simulink model "sampleModel307"  (R2021b)
settings: Solver=VariableStepAuto  StartTime=0.0  StopTime=10.0  RelTol=1e-3
libraries: simulink x3
settings Model: Creator=user  LastModifiedBy=user

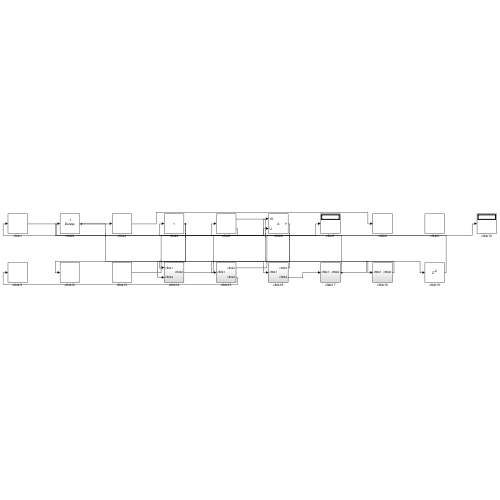
[thumbnail: Simulink's stored preview of the top-level diagram]
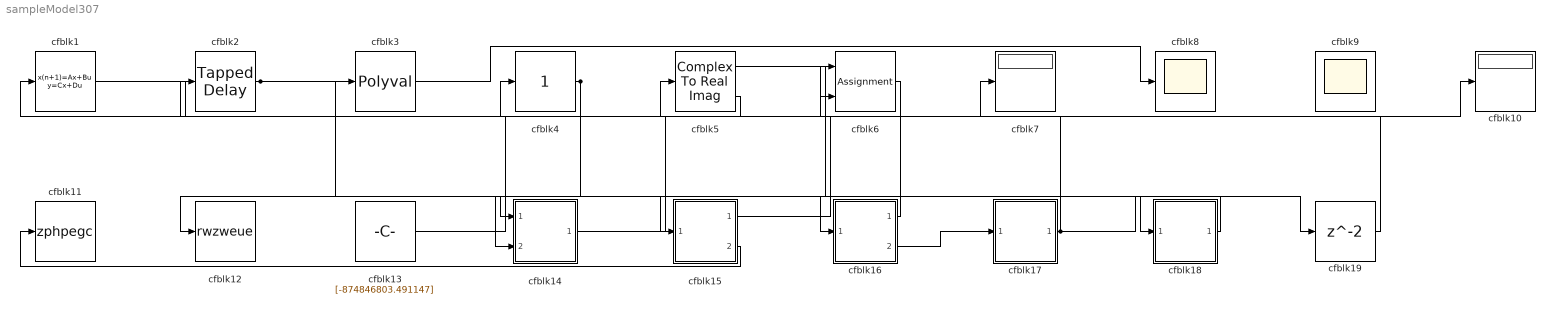
== system sampleModel307 ==
  cfblk1 : DiscreteStateSpace
  cfblk10 : Display
  cfblk11 : ToWorkspace  VariableName=zphpegc  SaveFormat=Timeseries  SampleTime=-1
  cfblk12 : ToWorkspace  VariableName=rwzweue  SaveFormat=Timeseries  SampleTime=-1
  cfblk13 : Constant  Value=[-874846803.491147]  SampleTime=1
  cfblk14 : Subsystem
  cfblk15 : Subsystem
  cfblk16 : Subsystem
  cfblk17 : Subsystem
  cfblk18 : Subsystem
  cfblk19 : Delay  SampleTime=1
  cfblk2 : simulink/Discrete/Tapped Delay  vinit=0.0  samptime=-1  NumDelays=1  DelayOrder=Oldest  includeCurrent=off
  cfblk3 : Polyval  Coefs=[ +2.081618890e-019, -1.441693666e-014, +4.719686976e-010, -8.536869453e-006, +1.621573104e-001, -8.087801117e+001 ]
  cfblk4 : simulink/Math Operations/Slider Gain  gain=1  low=0  high=2
  cfblk5 : ComplexToRealImag
  cfblk6 : Assignment  DiagnosticForDimensions=Warning  IndexOptions=Index vector (dialog)  Indices=1  OutputSizes=1
  cfblk7 : Display
  cfblk8 : Scope
  cfblk9 : Scope
      settings: Floating=on
  wires:
  cfblk4/1 -> cfblk12/1, cfblk14/2(cfblk4)
  cfblk14/1(cfblk2) -> cfblk10/1
  cfblk17/1(cfblk2) -> cfblk4/1, cfblk19/1
  cfblk5/1 -> cfblk18/1(cfblk1)
  cfblk16/1(cfblk2) -> cfblk5/1
  cfblk15/1(cfblk2) -> cfblk7/1
  cfblk5/2 -> cfblk1/1
  cfblk3/1 -> cfblk8/1
  cfblk15/2(cfblk4) -> cfblk11/1
  cfblk13/1 -> cfblk6/1
  cfblk2/1 -> cfblk3/1, cfblk16/1(cfblk1)
  cfblk1/1 -> cfblk6/2
  cfblk6/1 -> cfblk15/1(cfblk1)
  cfblk18/1(cfblk2) -> cfblk14/1(cfblk1)
  cfblk16/2(cfblk4) -> cfblk17/1(cfblk1)
  cfblk19/1 -> cfblk2/1

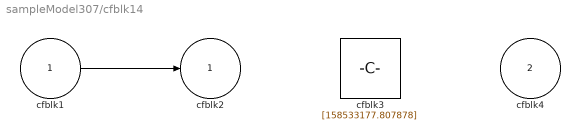
== system sampleModel307/cfblk14 ==
  cfblk1 : Inport
  cfblk4 : Inport  Port=2
  cfblk3 : Constant  Value=[158533177.807878]  SampleTime=1
  cfblk2 : Outport
  wires:
  cfblk1/1 -> cfblk2/1

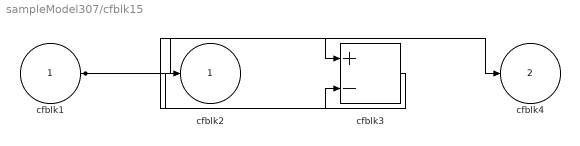
== system sampleModel307/cfblk15 ==
  cfblk1 : Inport
  cfblk3 : Sum  Inputs=+-
  cfblk2 : Outport
  cfblk4 : Outport  Port=2
  wires:
  cfblk1/1 -> cfblk4/1, cfblk3/1, cfblk3/2
  cfblk3/1 -> cfblk2/1

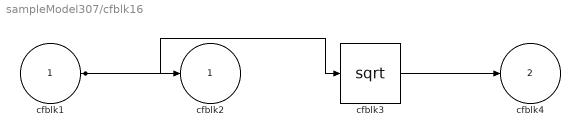
== system sampleModel307/cfblk16 ==
  cfblk1 : Inport
  cfblk3 : Sqrt  SaturateOnIntegerOverflow=on
  cfblk2 : Outport
  cfblk4 : Outport  Port=2
  wires:
  cfblk1/1 -> cfblk2/1, cfblk3/1
  cfblk3/1 -> cfblk4/1

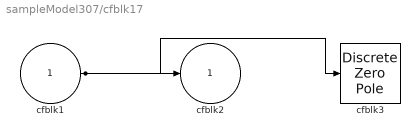
== system sampleModel307/cfblk17 ==
  cfblk1 : Inport
  cfblk3 : DiscreteZeroPole  Poles=[0 0.5]  Gain=1
  cfblk2 : Outport
  wires:
  cfblk1/1 -> cfblk2/1, cfblk3/1

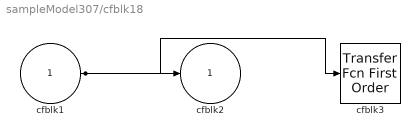
== system sampleModel307/cfblk18 ==
  cfblk1 : Inport
  cfblk3 : simulink/Discrete/Transfer Fcn First Order  PoleZ=0.95  ICPrevOutput=0.0  DoSatur=off
  cfblk2 : Outport
  wires:
  cfblk1/1 -> cfblk2/1, cfblk3/1
